simulink model "TST_Rail_MonMeUn"  (R2016b)
settings: Solver=FixedStepDiscrete  StartTime=0.0  StopTime=simTime  FixedStep=sampleTime  RelTol=1e-3
values from neighbouring files (symbols this model uses):
  testCase = 1    [initTST_Rail_MonMeUn_001.m]    (also in initTST_Rail_MonMeUn_002.m = 2; initTST_Rail_MonMeUn_003.m = 3; initTST_Rail_MonMeUn_004.m = 4; initTST_Rail_MonMeUn_005.m = 5)
libraries: simulink x91, UnitTest_Lib x81
(part 4 of 5)

== system TST_Rail_MonMeUn/simulationInput/testSignals_R005 ==
  BC : BusCreator  Inputs=40
  spec_APP_r : FromWorkspace  VariableName=testSig_APP_r  Interpolate=off  OutputAfterFinalValue=Holding final value
  spec_DFC_RailMeUn0_DSM : FromWorkspace  VariableName=testSig_DFC_RailMeUn0_DSM  Interpolate=off  OutputAfterFinalValue=Holding final value
  spec_DFC_RailMeUn10_DSM : FromWorkspace  VariableName=testSig_DFC_RailMeUn10_DSM  Interpolate=off  OutputAfterFinalValue=Holding final value
  spec_DFC_RailMeUn22_DSM : FromWorkspace  VariableName=testSig_DFC_RailMeUn22_DSM  Interpolate=off  OutputAfterFinalValue=Holding final value
  spec_DFC_RailMeUn2_DSM : FromWorkspace  VariableName=testSig_DFC_RailMeUn2_DSM  Interpolate=off  OutputAfterFinalValue=Holding final value
  spec_DFC_RailMeUn3_DSM : FromWorkspace  VariableName=testSig_DFC_RailMeUn3_DSM  Interpolate=off  OutputAfterFinalValue=Holding final value
  spec_DFC_RailMeUn42_DSM : FromWorkspace  VariableName=testSig_DFC_RailMeUn42_DSM  Interpolate=off  OutputAfterFinalValue=Holding final value
  spec_DFC_RailMeUn4_DSM : FromWorkspace  VariableName=testSig_DFC_RailMeUn4_DSM  Interpolate=off  OutputAfterFinalValue=Holding final value
  spec_DFC_RailMeUn7_DSM : FromWorkspace  VariableName=testSig_DFC_RailMeUn7_DSM  Interpolate=off  OutputAfterFinalValue=Holding final value
  spec_DFC_RailMeUn8_DSM : FromWorkspace  VariableName=testSig_DFC_RailMeUn8_DSM  Interpolate=off  OutputAfterFinalValue=Holding final value
  spec_DSM_bRailMeUn0Blk : FromWorkspace  VariableName=testSig_DSM_bRailMeUn0Blk  Interpolate=off  OutputAfterFinalValue=Holding final value
  spec_DSM_bRailMeUn0Rls : FromWorkspace  VariableName=testSig_DSM_bRailMeUn0Rls  Interpolate=off  OutputAfterFinalValue=Holding final value
  spec_DSM_bRailMeUn10Blk : FromWorkspace  VariableName=testSig_DSM_bRailMeUn10Blk  Interpolate=off  OutputAfterFinalValue=Holding final value
  spec_DSM_bRailMeUn10Rls : FromWorkspace  VariableName=testSig_DSM_bRailMeUn10Rls  Interpolate=off  OutputAfterFinalValue=Holding final value
  spec_DSM_bRailMeUn22Blk : FromWorkspace  VariableName=testSig_DSM_bRailMeUn22Blk  Interpolate=off  OutputAfterFinalValue=Holding final value
  spec_DSM_bRailMeUn22Rls : FromWorkspace  VariableName=testSig_DSM_bRailMeUn22Rls  Interpolate=off  OutputAfterFinalValue=Holding final value
  spec_DSM_bRailMeUn2Blk : FromWorkspace  VariableName=testSig_DSM_bRailMeUn2Blk  Interpolate=off  OutputAfterFinalValue=Holding final value
  spec_DSM_bRailMeUn2Rls : FromWorkspace  VariableName=testSig_DSM_bRailMeUn2Rls  Interpolate=off  OutputAfterFinalValue=Holding final value
  spec_DSM_bRailMeUn3Blk : FromWorkspace  VariableName=testSig_DSM_bRailMeUn3Blk  Interpolate=off  OutputAfterFinalValue=Holding final value
  spec_DSM_bRailMeUn3Rls : FromWorkspace  VariableName=testSig_DSM_bRailMeUn3Rls  Interpolate=off  OutputAfterFinalValue=Holding final value
  spec_DSM_bRailMeUn42Blk : FromWorkspace  VariableName=testSig_DSM_bRailMeUn42Blk  Interpolate=off  OutputAfterFinalValue=Holding final value
  spec_DSM_bRailMeUn42Rls : FromWorkspace  VariableName=testSig_DSM_bRailMeUn42Rls  Interpolate=off  OutputAfterFinalValue=Holding final value
  spec_DSM_bRailMeUn4Blk : FromWorkspace  VariableName=testSig_DSM_bRailMeUn4Blk  Interpolate=off  OutputAfterFinalValue=Holding final value
  spec_DSM_bRailMeUn4Rls : FromWorkspace  VariableName=testSig_DSM_bRailMeUn4Rls  Interpolate=off  OutputAfterFinalValue=Holding final value
  spec_DSM_bRailMeUn7Blk : FromWorkspace  VariableName=testSig_DSM_bRailMeUn7Blk  Interpolate=off  OutputAfterFinalValue=Holding final value
  spec_DSM_bRailMeUn7Rls : FromWorkspace  VariableName=testSig_DSM_bRailMeUn7Rls  Interpolate=off  OutputAfterFinalValue=Holding final value
  spec_DSM_bRailMeUn8Blk : FromWorkspace  VariableName=testSig_DSM_bRailMeUn8Blk  Interpolate=off  OutputAfterFinalValue=Holding final value
  spec_DSM_bRailMeUn8Rls : FromWorkspace  VariableName=testSig_DSM_bRailMeUn8Rls  Interpolate=off  OutputAfterFinalValue=Holding final value
  spec_Epm_nEng : FromWorkspace  VariableName=testSig_Epm_nEng  Interpolate=off  OutputAfterFinalValue=Holding final value
  spec_FuelT_tFlSys : FromWorkspace  VariableName=testSig_FuelT_tFlSys  Interpolate=off  OutputAfterFinalValue=Holding final value
  spec_InjCtl_qSetUnBal : FromWorkspace  VariableName=testSig_InjCtl_qSetUnBal  Interpolate=off  OutputAfterFinalValue=Holding final value
  spec_MeUn_dvolSet : FromWorkspace  VariableName=testSig_MeUn_dvolSet  Interpolate=off  OutputAfterFinalValue=Holding final value
  spec_MeUn_dvolSetAdapt : FromWorkspace  VariableName=testSig_MeUn_dvolSetAdapt  Interpolate=off  OutputAfterFinalValue=Holding final value
  spec_PthSet_stOvrRun : FromWorkspace  VariableName=testSig_PthSet_stOvrRun  Interpolate=off  OutputAfterFinalValue=Holding final value
  spec_RailP_pFlt : FromWorkspace  VariableName=testSig_RailP_pFlt  Interpolate=off  OutputAfterFinalValue=Holding final value
  spec_Rail_dvolDemSysMax : FromWorkspace  VariableName=testSig_Rail_dvolDemSysMax  Interpolate=off  OutputAfterFinalValue=Holding final value
  spec_Rail_dvolMeUnCtlUpLim : FromWorkspace  VariableName=testSig_Rail_dvolMeUnCtlUpLim  Interpolate=off  OutputAfterFinalValue=Holding final value
  spec_Rail_pDvt : FromWorkspace  VariableName=testSig_Rail_pDvt  Interpolate=off  OutputAfterFinalValue=Holding final value
  spec_Rail_pSetPoint : FromWorkspace  VariableName=testSig_Rail_pSetPoint  Interpolate=off  OutputAfterFinalValue=Holding final value
  spec_Rail_stCtlLoop : FromWorkspace  VariableName=testSig_Rail_stCtlLoop  Interpolate=off  OutputAfterFinalValue=Holding final value
  testSignals : Outport
  wires:
  BC/1 -> testSignals/1
  spec_Rail_pDvt/1 -> BC/1  "testSig_Rail_pDvt"
  spec_Epm_nEng/1 -> BC/2  "testSig_Epm_nEng"
  spec_MeUn_dvolSet/1 -> BC/3  "testSig_MeUn_dvolSet"
  spec_Rail_dvolMeUnCtlUpLim/1 -> BC/4  "testSig_Rail_dvolMeUnCtlUpLim"
  spec_Rail_stCtlLoop/1 -> BC/5  "testSig_Rail_stCtlLoop"
  spec_InjCtl_qSetUnBal/1 -> BC/6  "testSig_InjCtl_qSetUnBal"
  spec_FuelT_tFlSys/1 -> BC/7  "testSig_FuelT_tFlSys"
  spec_Rail_pSetPoint/1 -> BC/8  "testSig_Rail_pSetPoint"
  spec_Rail_dvolDemSysMax/1 -> BC/9  "testSig_Rail_dvolDemSysMax"
  spec_RailP_pFlt/1 -> BC/10  "testSig_RailP_pFlt"
  spec_MeUn_dvolSetAdapt/1 -> BC/11  "testSig_MeUn_dvolSetAdapt"
  spec_PthSet_stOvrRun/1 -> BC/12  "testSig_PthSet_stOvrRun"
  spec_APP_r/1 -> BC/13  "testSig_APP_r"
  spec_DSM_bRailMeUn0Rls/1 -> BC/14  "testSig_DSM_bRailMeUn0Rls"
  spec_DSM_bRailMeUn0Blk/1 -> BC/15  "testSig_DSM_bRailMeUn0Blk"
  spec_DSM_bRailMeUn2Rls/1 -> BC/16  "testSig_DSM_bRailMeUn2Rls"
  spec_DSM_bRailMeUn2Blk/1 -> BC/17  "testSig_DSM_bRailMeUn2Blk"
  spec_DSM_bRailMeUn22Rls/1 -> BC/18  "testSig_DSM_bRailMeUn22Rls"
  spec_DSM_bRailMeUn22Blk/1 -> BC/19  "testSig_DSM_bRailMeUn22Blk"
  spec_DSM_bRailMeUn3Rls/1 -> BC/20  "testSig_DSM_bRailMeUn3Rls"
  spec_DSM_bRailMeUn3Blk/1 -> BC/21  "testSig_DSM_bRailMeUn3Blk"
  spec_DSM_bRailMeUn4Rls/1 -> BC/22  "testSig_DSM_bRailMeUn4Rls"
  spec_DSM_bRailMeUn4Blk/1 -> BC/23  "testSig_DSM_bRailMeUn4Blk"
  spec_DSM_bRailMeUn42Rls/1 -> BC/24  "testSig_DSM_bRailMeUn42Rls"
  spec_DSM_bRailMeUn42Blk/1 -> BC/25  "testSig_DSM_bRailMeUn42Blk"
  spec_DSM_bRailMeUn7Rls/1 -> BC/26  "testSig_DSM_bRailMeUn7Rls"
  spec_DSM_bRailMeUn7Blk/1 -> BC/27  "testSig_DSM_bRailMeUn7Blk"
  spec_DSM_bRailMeUn8Rls/1 -> BC/28  "testSig_DSM_bRailMeUn8Rls"
  spec_DSM_bRailMeUn8Blk/1 -> BC/29  "testSig_DSM_bRailMeUn8Blk"
  spec_DSM_bRailMeUn10Rls/1 -> BC/30  "testSig_DSM_bRailMeUn10Rls"
  spec_DSM_bRailMeUn10Blk/1 -> BC/31  "testSig_DSM_bRailMeUn10Blk"
  spec_DFC_RailMeUn0_DSM/1 -> BC/32  "testSig_DFC_RailMeUn0_DSM"
  spec_DFC_RailMeUn2_DSM/1 -> BC/33  "testSig_DFC_RailMeUn2_DSM"
  spec_DFC_RailMeUn22_DSM/1 -> BC/34  "testSig_DFC_RailMeUn22_DSM"
  spec_DFC_RailMeUn3_DSM/1 -> BC/35  "testSig_DFC_RailMeUn3_DSM"
  spec_DFC_RailMeUn4_DSM/1 -> BC/36  "testSig_DFC_RailMeUn4_DSM"
  spec_DFC_RailMeUn42_DSM/1 -> BC/37  "testSig_DFC_RailMeUn42_DSM"
  spec_DFC_RailMeUn7_DSM/1 -> BC/38  "testSig_DFC_RailMeUn7_DSM"
  spec_DFC_RailMeUn8_DSM/1 -> BC/39  "testSig_DFC_RailMeUn8_DSM"
  spec_DFC_RailMeUn10_DSM/1 -> BC/40  "testSig_DFC_RailMeUn10_DSM"

== system TST_Rail_MonMeUn/simulationInput/testSignals_R006 ==
  BC : BusCreator  Inputs=40
  spec_APP_r : FromWorkspace  VariableName=testSig_APP_r  Interpolate=off  OutputAfterFinalValue=Holding final value
  spec_DFC_RailMeUn0_DSM : FromWorkspace  VariableName=testSig_DFC_RailMeUn0_DSM  Interpolate=off  OutputAfterFinalValue=Holding final value
  spec_DFC_RailMeUn10_DSM : FromWorkspace  VariableName=testSig_DFC_RailMeUn10_DSM  Interpolate=off  OutputAfterFinalValue=Holding final value
  spec_DFC_RailMeUn22_DSM : FromWorkspace  VariableName=testSig_DFC_RailMeUn22_DSM  Interpolate=off  OutputAfterFinalValue=Holding final value
  spec_DFC_RailMeUn2_DSM : FromWorkspace  VariableName=testSig_DFC_RailMeUn2_DSM  Interpolate=off  OutputAfterFinalValue=Holding final value
  spec_DFC_RailMeUn3_DSM : FromWorkspace  VariableName=testSig_DFC_RailMeUn3_DSM  Interpolate=off  OutputAfterFinalValue=Holding final value
  spec_DFC_RailMeUn42_DSM : FromWorkspace  VariableName=testSig_DFC_RailMeUn42_DSM  Interpolate=off  OutputAfterFinalValue=Holding final value
  spec_DFC_RailMeUn4_DSM : FromWorkspace  VariableName=testSig_DFC_RailMeUn4_DSM  Interpolate=off  OutputAfterFinalValue=Holding final value
  spec_DFC_RailMeUn7_DSM : FromWorkspace  VariableName=testSig_DFC_RailMeUn7_DSM  Interpolate=off  OutputAfterFinalValue=Holding final value
  spec_DFC_RailMeUn8_DSM : FromWorkspace  VariableName=testSig_DFC_RailMeUn8_DSM  Interpolate=off  OutputAfterFinalValue=Holding final value
  spec_DSM_bRailMeUn0Blk : FromWorkspace  VariableName=testSig_DSM_bRailMeUn0Blk  Interpolate=off  OutputAfterFinalValue=Holding final value
  spec_DSM_bRailMeUn0Rls : FromWorkspace  VariableName=testSig_DSM_bRailMeUn0Rls  Interpolate=off  OutputAfterFinalValue=Holding final value
  spec_DSM_bRailMeUn10Blk : FromWorkspace  VariableName=testSig_DSM_bRailMeUn10Blk  Interpolate=off  OutputAfterFinalValue=Holding final value
  spec_DSM_bRailMeUn10Rls : FromWorkspace  VariableName=testSig_DSM_bRailMeUn10Rls  Interpolate=off  OutputAfterFinalValue=Holding final value
  spec_DSM_bRailMeUn22Blk : FromWorkspace  VariableName=testSig_DSM_bRailMeUn22Blk  Interpolate=off  OutputAfterFinalValue=Holding final value
  spec_DSM_bRailMeUn22Rls : FromWorkspace  VariableName=testSig_DSM_bRailMeUn22Rls  Interpolate=off  OutputAfterFinalValue=Holding final value
  spec_DSM_bRailMeUn2Blk : FromWorkspace  VariableName=testSig_DSM_bRailMeUn2Blk  Interpolate=off  OutputAfterFinalValue=Holding final value
  spec_DSM_bRailMeUn2Rls : FromWorkspace  VariableName=testSig_DSM_bRailMeUn2Rls  Interpolate=off  OutputAfterFinalValue=Holding final value
  spec_DSM_bRailMeUn3Blk : FromWorkspace  VariableName=testSig_DSM_bRailMeUn3Blk  Interpolate=off  OutputAfterFinalValue=Holding final value
  spec_DSM_bRailMeUn3Rls : FromWorkspace  VariableName=testSig_DSM_bRailMeUn3Rls  Interpolate=off  OutputAfterFinalValue=Holding final value
  spec_DSM_bRailMeUn42Blk : FromWorkspace  VariableName=testSig_DSM_bRailMeUn42Blk  Interpolate=off  OutputAfterFinalValue=Holding final value
  spec_DSM_bRailMeUn42Rls : FromWorkspace  VariableName=testSig_DSM_bRailMeUn42Rls  Interpolate=off  OutputAfterFinalValue=Holding final value
  spec_DSM_bRailMeUn4Blk : FromWorkspace  VariableName=testSig_DSM_bRailMeUn4Blk  Interpolate=off  OutputAfterFinalValue=Holding final value
  spec_DSM_bRailMeUn4Rls : FromWorkspace  VariableName=testSig_DSM_bRailMeUn4Rls  Interpolate=off  OutputAfterFinalValue=Holding final value
  spec_DSM_bRailMeUn7Blk : FromWorkspace  VariableName=testSig_DSM_bRailMeUn7Blk  Interpolate=off  OutputAfterFinalValue=Holding final value
  spec_DSM_bRailMeUn7Rls : FromWorkspace  VariableName=testSig_DSM_bRailMeUn7Rls  Interpolate=off  OutputAfterFinalValue=Holding final value
  spec_DSM_bRailMeUn8Blk : FromWorkspace  VariableName=testSig_DSM_bRailMeUn8Blk  Interpolate=off  OutputAfterFinalValue=Holding final value
  spec_DSM_bRailMeUn8Rls : FromWorkspace  VariableName=testSig_DSM_bRailMeUn8Rls  Interpolate=off  OutputAfterFinalValue=Holding final value
  spec_Epm_nEng : FromWorkspace  VariableName=testSig_Epm_nEng  Interpolate=off  OutputAfterFinalValue=Holding final value
  spec_FuelT_tFlSys : FromWorkspace  VariableName=testSig_FuelT_tFlSys  Interpolate=off  OutputAfterFinalValue=Holding final value
  spec_InjCtl_qSetUnBal : FromWorkspace  VariableName=testSig_InjCtl_qSetUnBal  Interpolate=off  OutputAfterFinalValue=Holding final value
  spec_MeUn_dvolSet : FromWorkspace  VariableName=testSig_MeUn_dvolSet  Interpolate=off  OutputAfterFinalValue=Holding final value
  spec_MeUn_dvolSetAdapt : FromWorkspace  VariableName=testSig_MeUn_dvolSetAdapt  Interpolate=off  OutputAfterFinalValue=Holding final value
  spec_PthSet_stOvrRun : FromWorkspace  VariableName=testSig_PthSet_stOvrRun  Interpolate=off  OutputAfterFinalValue=Holding final value
  spec_RailP_pFlt : FromWorkspace  VariableName=testSig_RailP_pFlt  Interpolate=off  OutputAfterFinalValue=Holding final value
  spec_Rail_dvolDemSysMax : FromWorkspace  VariableName=testSig_Rail_dvolDemSysMax  Interpolate=off  OutputAfterFinalValue=Holding final value
  spec_Rail_dvolMeUnCtlUpLim : FromWorkspace  VariableName=testSig_Rail_dvolMeUnCtlUpLim  Interpolate=off  OutputAfterFinalValue=Holding final value
  spec_Rail_pDvt : FromWorkspace  VariableName=testSig_Rail_pDvt  Interpolate=off  OutputAfterFinalValue=Holding final value
  spec_Rail_pSetPoint : FromWorkspace  VariableName=testSig_Rail_pSetPoint  Interpolate=off  OutputAfterFinalValue=Holding final value
  spec_Rail_stCtlLoop : FromWorkspace  VariableName=testSig_Rail_stCtlLoop  Interpolate=off  OutputAfterFinalValue=Holding final value
  testSignals : Outport
  wires:
  BC/1 -> testSignals/1
  spec_Rail_pDvt/1 -> BC/1  "testSig_Rail_pDvt"
  spec_Epm_nEng/1 -> BC/2  "testSig_Epm_nEng"
  spec_MeUn_dvolSet/1 -> BC/3  "testSig_MeUn_dvolSet"
  spec_Rail_dvolMeUnCtlUpLim/1 -> BC/4  "testSig_Rail_dvolMeUnCtlUpLim"
  spec_Rail_stCtlLoop/1 -> BC/5  "testSig_Rail_stCtlLoop"
  spec_InjCtl_qSetUnBal/1 -> BC/6  "testSig_InjCtl_qSetUnBal"
  spec_FuelT_tFlSys/1 -> BC/7  "testSig_FuelT_tFlSys"
  spec_Rail_pSetPoint/1 -> BC/8  "testSig_Rail_pSetPoint"
  spec_Rail_dvolDemSysMax/1 -> BC/9  "testSig_Rail_dvolDemSysMax"
  spec_RailP_pFlt/1 -> BC/10  "testSig_RailP_pFlt"
  spec_MeUn_dvolSetAdapt/1 -> BC/11  "testSig_MeUn_dvolSetAdapt"
  spec_PthSet_stOvrRun/1 -> BC/12  "testSig_PthSet_stOvrRun"
  spec_APP_r/1 -> BC/13  "testSig_APP_r"
  spec_DSM_bRailMeUn0Rls/1 -> BC/14  "testSig_DSM_bRailMeUn0Rls"
  spec_DSM_bRailMeUn0Blk/1 -> BC/15  "testSig_DSM_bRailMeUn0Blk"
  spec_DSM_bRailMeUn2Rls/1 -> BC/16  "testSig_DSM_bRailMeUn2Rls"
  spec_DSM_bRailMeUn2Blk/1 -> BC/17  "testSig_DSM_bRailMeUn2Blk"
  spec_DSM_bRailMeUn22Rls/1 -> BC/18  "testSig_DSM_bRailMeUn22Rls"
  spec_DSM_bRailMeUn22Blk/1 -> BC/19  "testSig_DSM_bRailMeUn22Blk"
  spec_DSM_bRailMeUn3Rls/1 -> BC/20  "testSig_DSM_bRailMeUn3Rls"
  spec_DSM_bRailMeUn3Blk/1 -> BC/21  "testSig_DSM_bRailMeUn3Blk"
  spec_DSM_bRailMeUn4Rls/1 -> BC/22  "testSig_DSM_bRailMeUn4Rls"
  spec_DSM_bRailMeUn4Blk/1 -> BC/23  "testSig_DSM_bRailMeUn4Blk"
  spec_DSM_bRailMeUn42Rls/1 -> BC/24  "testSig_DSM_bRailMeUn42Rls"
  spec_DSM_bRailMeUn42Blk/1 -> BC/25  "testSig_DSM_bRailMeUn42Blk"
  spec_DSM_bRailMeUn7Rls/1 -> BC/26  "testSig_DSM_bRailMeUn7Rls"
  spec_DSM_bRailMeUn7Blk/1 -> BC/27  "testSig_DSM_bRailMeUn7Blk"
  spec_DSM_bRailMeUn8Rls/1 -> BC/28  "testSig_DSM_bRailMeUn8Rls"
  spec_DSM_bRailMeUn8Blk/1 -> BC/29  "testSig_DSM_bRailMeUn8Blk"
  spec_DSM_bRailMeUn10Rls/1 -> BC/30  "testSig_DSM_bRailMeUn10Rls"
  spec_DSM_bRailMeUn10Blk/1 -> BC/31  "testSig_DSM_bRailMeUn10Blk"
  spec_DFC_RailMeUn0_DSM/1 -> BC/32  "testSig_DFC_RailMeUn0_DSM"
  spec_DFC_RailMeUn2_DSM/1 -> BC/33  "testSig_DFC_RailMeUn2_DSM"
  spec_DFC_RailMeUn22_DSM/1 -> BC/34  "testSig_DFC_RailMeUn22_DSM"
  spec_DFC_RailMeUn3_DSM/1 -> BC/35  "testSig_DFC_RailMeUn3_DSM"
  spec_DFC_RailMeUn4_DSM/1 -> BC/36  "testSig_DFC_RailMeUn4_DSM"
  spec_DFC_RailMeUn42_DSM/1 -> BC/37  "testSig_DFC_RailMeUn42_DSM"
  spec_DFC_RailMeUn7_DSM/1 -> BC/38  "testSig_DFC_RailMeUn7_DSM"
  spec_DFC_RailMeUn8_DSM/1 -> BC/39  "testSig_DFC_RailMeUn8_DSM"
  spec_DFC_RailMeUn10_DSM/1 -> BC/40  "testSig_DFC_RailMeUn10_DSM"

== system TST_Rail_MonMeUn/simulationInput/testSignals_R007 ==
  BC : BusCreator  Inputs=40
  spec_APP_r : FromWorkspace  VariableName=testSig_APP_r  Interpolate=off  OutputAfterFinalValue=Holding final value
  spec_DFC_RailMeUn0_DSM : FromWorkspace  VariableName=testSig_DFC_RailMeUn0_DSM  Interpolate=off  OutputAfterFinalValue=Holding final value
  spec_DFC_RailMeUn10_DSM : FromWorkspace  VariableName=testSig_DFC_RailMeUn10_DSM  Interpolate=off  OutputAfterFinalValue=Holding final value
  spec_DFC_RailMeUn22_DSM : FromWorkspace  VariableName=testSig_DFC_RailMeUn22_DSM  Interpolate=off  OutputAfterFinalValue=Holding final value
  spec_DFC_RailMeUn2_DSM : FromWorkspace  VariableName=testSig_DFC_RailMeUn2_DSM  Interpolate=off  OutputAfterFinalValue=Holding final value
  spec_DFC_RailMeUn3_DSM : FromWorkspace  VariableName=testSig_DFC_RailMeUn3_DSM  Interpolate=off  OutputAfterFinalValue=Holding final value
  spec_DFC_RailMeUn42_DSM : FromWorkspace  VariableName=testSig_DFC_RailMeUn42_DSM  Interpolate=off  OutputAfterFinalValue=Holding final value
  spec_DFC_RailMeUn4_DSM : FromWorkspace  VariableName=testSig_DFC_RailMeUn4_DSM  Interpolate=off  OutputAfterFinalValue=Holding final value
  spec_DFC_RailMeUn7_DSM : FromWorkspace  VariableName=testSig_DFC_RailMeUn7_DSM  Interpolate=off  OutputAfterFinalValue=Holding final value
  spec_DFC_RailMeUn8_DSM : FromWorkspace  VariableName=testSig_DFC_RailMeUn8_DSM  Interpolate=off  OutputAfterFinalValue=Holding final value
  spec_DSM_bRailMeUn0Blk : FromWorkspace  VariableName=testSig_DSM_bRailMeUn0Blk  Interpolate=off  OutputAfterFinalValue=Holding final value
  spec_DSM_bRailMeUn0Rls : FromWorkspace  VariableName=testSig_DSM_bRailMeUn0Rls  Interpolate=off  OutputAfterFinalValue=Holding final value
  spec_DSM_bRailMeUn10Blk : FromWorkspace  VariableName=testSig_DSM_bRailMeUn10Blk  Interpolate=off  OutputAfterFinalValue=Holding final value
  spec_DSM_bRailMeUn10Rls : FromWorkspace  VariableName=testSig_DSM_bRailMeUn10Rls  Interpolate=off  OutputAfterFinalValue=Holding final value
  spec_DSM_bRailMeUn22Blk : FromWorkspace  VariableName=testSig_DSM_bRailMeUn22Blk  Interpolate=off  OutputAfterFinalValue=Holding final value
  spec_DSM_bRailMeUn22Rls : FromWorkspace  VariableName=testSig_DSM_bRailMeUn22Rls  Interpolate=off  OutputAfterFinalValue=Holding final value
  spec_DSM_bRailMeUn2Blk : FromWorkspace  VariableName=testSig_DSM_bRailMeUn2Blk  Interpolate=off  OutputAfterFinalValue=Holding final value
  spec_DSM_bRailMeUn2Rls : FromWorkspace  VariableName=testSig_DSM_bRailMeUn2Rls  Interpolate=off  OutputAfterFinalValue=Holding final value
  spec_DSM_bRailMeUn3Blk : FromWorkspace  VariableName=testSig_DSM_bRailMeUn3Blk  Interpolate=off  OutputAfterFinalValue=Holding final value
  spec_DSM_bRailMeUn3Rls : FromWorkspace  VariableName=testSig_DSM_bRailMeUn3Rls  Interpolate=off  OutputAfterFinalValue=Holding final value
  spec_DSM_bRailMeUn42Blk : FromWorkspace  VariableName=testSig_DSM_bRailMeUn42Blk  Interpolate=off  OutputAfterFinalValue=Holding final value
  spec_DSM_bRailMeUn42Rls : FromWorkspace  VariableName=testSig_DSM_bRailMeUn42Rls  Interpolate=off  OutputAfterFinalValue=Holding final value
  spec_DSM_bRailMeUn4Blk : FromWorkspace  VariableName=testSig_DSM_bRailMeUn4Blk  Interpolate=off  OutputAfterFinalValue=Holding final value
  spec_DSM_bRailMeUn4Rls : FromWorkspace  VariableName=testSig_DSM_bRailMeUn4Rls  Interpolate=off  OutputAfterFinalValue=Holding final value
  spec_DSM_bRailMeUn7Blk : FromWorkspace  VariableName=testSig_DSM_bRailMeUn7Blk  Interpolate=off  OutputAfterFinalValue=Holding final value
  spec_DSM_bRailMeUn7Rls : FromWorkspace  VariableName=testSig_DSM_bRailMeUn7Rls  Interpolate=off  OutputAfterFinalValue=Holding final value
  spec_DSM_bRailMeUn8Blk : FromWorkspace  VariableName=testSig_DSM_bRailMeUn8Blk  Interpolate=off  OutputAfterFinalValue=Holding final value
  spec_DSM_bRailMeUn8Rls : FromWorkspace  VariableName=testSig_DSM_bRailMeUn8Rls  Interpolate=off  OutputAfterFinalValue=Holding final value
  spec_Epm_nEng : FromWorkspace  VariableName=testSig_Epm_nEng  Interpolate=off  OutputAfterFinalValue=Holding final value
  spec_FuelT_tFlSys : FromWorkspace  VariableName=testSig_FuelT_tFlSys  Interpolate=off  OutputAfterFinalValue=Holding final value
  spec_InjCtl_qSetUnBal : FromWorkspace  VariableName=testSig_InjCtl_qSetUnBal  Interpolate=off  OutputAfterFinalValue=Holding final value
  spec_MeUn_dvolSet : FromWorkspace  VariableName=testSig_MeUn_dvolSet  Interpolate=off  OutputAfterFinalValue=Holding final value
  spec_MeUn_dvolSetAdapt : FromWorkspace  VariableName=testSig_MeUn_dvolSetAdapt  Interpolate=off  OutputAfterFinalValue=Holding final value
  spec_PthSet_stOvrRun : FromWorkspace  VariableName=testSig_PthSet_stOvrRun  Interpolate=off  OutputAfterFinalValue=Holding final value
  spec_RailP_pFlt : FromWorkspace  VariableName=testSig_RailP_pFlt  Interpolate=off  OutputAfterFinalValue=Holding final value
  spec_Rail_dvolDemSysMax : FromWorkspace  VariableName=testSig_Rail_dvolDemSysMax  Interpolate=off  OutputAfterFinalValue=Holding final value
  spec_Rail_dvolMeUnCtlUpLim : FromWorkspace  VariableName=testSig_Rail_dvolMeUnCtlUpLim  Interpolate=off  OutputAfterFinalValue=Holding final value
  spec_Rail_pDvt : FromWorkspace  VariableName=testSig_Rail_pDvt  Interpolate=off  OutputAfterFinalValue=Holding final value
  spec_Rail_pSetPoint : FromWorkspace  VariableName=testSig_Rail_pSetPoint  Interpolate=off  OutputAfterFinalValue=Holding final value
  spec_Rail_stCtlLoop : FromWorkspace  VariableName=testSig_Rail_stCtlLoop  Interpolate=off  OutputAfterFinalValue=Holding final value
  testSignals : Outport
  wires:
  BC/1 -> testSignals/1
  spec_Rail_pDvt/1 -> BC/1  "testSig_Rail_pDvt"
  spec_Epm_nEng/1 -> BC/2  "testSig_Epm_nEng"
  spec_MeUn_dvolSet/1 -> BC/3  "testSig_MeUn_dvolSet"
  spec_Rail_dvolMeUnCtlUpLim/1 -> BC/4  "testSig_Rail_dvolMeUnCtlUpLim"
  spec_Rail_stCtlLoop/1 -> BC/5  "testSig_Rail_stCtlLoop"
  spec_InjCtl_qSetUnBal/1 -> BC/6  "testSig_InjCtl_qSetUnBal"
  spec_FuelT_tFlSys/1 -> BC/7  "testSig_FuelT_tFlSys"
  spec_Rail_pSetPoint/1 -> BC/8  "testSig_Rail_pSetPoint"
  spec_Rail_dvolDemSysMax/1 -> BC/9  "testSig_Rail_dvolDemSysMax"
  spec_RailP_pFlt/1 -> BC/10  "testSig_RailP_pFlt"
  spec_MeUn_dvolSetAdapt/1 -> BC/11  "testSig_MeUn_dvolSetAdapt"
  spec_PthSet_stOvrRun/1 -> BC/12  "testSig_PthSet_stOvrRun"
  spec_APP_r/1 -> BC/13  "testSig_APP_r"
  spec_DSM_bRailMeUn0Rls/1 -> BC/14  "testSig_DSM_bRailMeUn0Rls"
  spec_DSM_bRailMeUn0Blk/1 -> BC/15  "testSig_DSM_bRailMeUn0Blk"
  spec_DSM_bRailMeUn2Rls/1 -> BC/16  "testSig_DSM_bRailMeUn2Rls"
  spec_DSM_bRailMeUn2Blk/1 -> BC/17  "testSig_DSM_bRailMeUn2Blk"
  spec_DSM_bRailMeUn22Rls/1 -> BC/18  "testSig_DSM_bRailMeUn22Rls"
  spec_DSM_bRailMeUn22Blk/1 -> BC/19  "testSig_DSM_bRailMeUn22Blk"
  spec_DSM_bRailMeUn3Rls/1 -> BC/20  "testSig_DSM_bRailMeUn3Rls"
  spec_DSM_bRailMeUn3Blk/1 -> BC/21  "testSig_DSM_bRailMeUn3Blk"
  spec_DSM_bRailMeUn4Rls/1 -> BC/22  "testSig_DSM_bRailMeUn4Rls"
  spec_DSM_bRailMeUn4Blk/1 -> BC/23  "testSig_DSM_bRailMeUn4Blk"
  spec_DSM_bRailMeUn42Rls/1 -> BC/24  "testSig_DSM_bRailMeUn42Rls"
  spec_DSM_bRailMeUn42Blk/1 -> BC/25  "testSig_DSM_bRailMeUn42Blk"
  spec_DSM_bRailMeUn7Rls/1 -> BC/26  "testSig_DSM_bRailMeUn7Rls"
  spec_DSM_bRailMeUn7Blk/1 -> BC/27  "testSig_DSM_bRailMeUn7Blk"
  spec_DSM_bRailMeUn8Rls/1 -> BC/28  "testSig_DSM_bRailMeUn8Rls"
  spec_DSM_bRailMeUn8Blk/1 -> BC/29  "testSig_DSM_bRailMeUn8Blk"
  spec_DSM_bRailMeUn10Rls/1 -> BC/30  "testSig_DSM_bRailMeUn10Rls"
  spec_DSM_bRailMeUn10Blk/1 -> BC/31  "testSig_DSM_bRailMeUn10Blk"
  spec_DFC_RailMeUn0_DSM/1 -> BC/32  "testSig_DFC_RailMeUn0_DSM"
  spec_DFC_RailMeUn2_DSM/1 -> BC/33  "testSig_DFC_RailMeUn2_DSM"
  spec_DFC_RailMeUn22_DSM/1 -> BC/34  "testSig_DFC_RailMeUn22_DSM"
  spec_DFC_RailMeUn3_DSM/1 -> BC/35  "testSig_DFC_RailMeUn3_DSM"
  spec_DFC_RailMeUn4_DSM/1 -> BC/36  "testSig_DFC_RailMeUn4_DSM"
  spec_DFC_RailMeUn42_DSM/1 -> BC/37  "testSig_DFC_RailMeUn42_DSM"
  spec_DFC_RailMeUn7_DSM/1 -> BC/38  "testSig_DFC_RailMeUn7_DSM"
  spec_DFC_RailMeUn8_DSM/1 -> BC/39  "testSig_DFC_RailMeUn8_DSM"
  spec_DFC_RailMeUn10_DSM/1 -> BC/40  "testSig_DFC_RailMeUn10_DSM"

== system TST_Rail_MonMeUn/simulationInput/testSignals_R008 ==
  BC : BusCreator  Inputs=40
  spec_APP_r : FromWorkspace  VariableName=testSig_APP_r  Interpolate=off  OutputAfterFinalValue=Holding final value
  spec_DFC_RailMeUn0_DSM : FromWorkspace  VariableName=testSig_DFC_RailMeUn0_DSM  Interpolate=off  OutputAfterFinalValue=Holding final value
  spec_DFC_RailMeUn10_DSM : FromWorkspace  VariableName=testSig_DFC_RailMeUn10_DSM  Interpolate=off  OutputAfterFinalValue=Holding final value
  spec_DFC_RailMeUn22_DSM : FromWorkspace  VariableName=testSig_DFC_RailMeUn22_DSM  Interpolate=off  OutputAfterFinalValue=Holding final value
  spec_DFC_RailMeUn2_DSM : FromWorkspace  VariableName=testSig_DFC_RailMeUn2_DSM  Interpolate=off  OutputAfterFinalValue=Holding final value
  spec_DFC_RailMeUn3_DSM : FromWorkspace  VariableName=testSig_DFC_RailMeUn3_DSM  Interpolate=off  OutputAfterFinalValue=Holding final value
  spec_DFC_RailMeUn42_DSM : FromWorkspace  VariableName=testSig_DFC_RailMeUn42_DSM  Interpolate=off  OutputAfterFinalValue=Holding final value
  spec_DFC_RailMeUn4_DSM : FromWorkspace  VariableName=testSig_DFC_RailMeUn4_DSM  Interpolate=off  OutputAfterFinalValue=Holding final value
  spec_DFC_RailMeUn7_DSM : FromWorkspace  VariableName=testSig_DFC_RailMeUn7_DSM  Interpolate=off  OutputAfterFinalValue=Holding final value
  spec_DFC_RailMeUn8_DSM : FromWorkspace  VariableName=testSig_DFC_RailMeUn8_DSM  Interpolate=off  OutputAfterFinalValue=Holding final value
  spec_DSM_bRailMeUn0Blk : FromWorkspace  VariableName=testSig_DSM_bRailMeUn0Blk  Interpolate=off  OutputAfterFinalValue=Holding final value
  spec_DSM_bRailMeUn0Rls : FromWorkspace  VariableName=testSig_DSM_bRailMeUn0Rls  Interpolate=off  OutputAfterFinalValue=Holding final value
  spec_DSM_bRailMeUn10Blk : FromWorkspace  VariableName=testSig_DSM_bRailMeUn10Blk  Interpolate=off  OutputAfterFinalValue=Holding final value
  spec_DSM_bRailMeUn10Rls : FromWorkspace  VariableName=testSig_DSM_bRailMeUn10Rls  Interpolate=off  OutputAfterFinalValue=Holding final value
  spec_DSM_bRailMeUn22Blk : FromWorkspace  VariableName=testSig_DSM_bRailMeUn22Blk  Interpolate=off  OutputAfterFinalValue=Holding final value
  spec_DSM_bRailMeUn22Rls : FromWorkspace  VariableName=testSig_DSM_bRailMeUn22Rls  Interpolate=off  OutputAfterFinalValue=Holding final value
  spec_DSM_bRailMeUn2Blk : FromWorkspace  VariableName=testSig_DSM_bRailMeUn2Blk  Interpolate=off  OutputAfterFinalValue=Holding final value
  spec_DSM_bRailMeUn2Rls : FromWorkspace  VariableName=testSig_DSM_bRailMeUn2Rls  Interpolate=off  OutputAfterFinalValue=Holding final value
  spec_DSM_bRailMeUn3Blk : FromWorkspace  VariableName=testSig_DSM_bRailMeUn3Blk  Interpolate=off  OutputAfterFinalValue=Holding final value
  spec_DSM_bRailMeUn3Rls : FromWorkspace  VariableName=testSig_DSM_bRailMeUn3Rls  Interpolate=off  OutputAfterFinalValue=Holding final value
  spec_DSM_bRailMeUn42Blk : FromWorkspace  VariableName=testSig_DSM_bRailMeUn42Blk  Interpolate=off  OutputAfterFinalValue=Holding final value
  spec_DSM_bRailMeUn42Rls : FromWorkspace  VariableName=testSig_DSM_bRailMeUn42Rls  Interpolate=off  OutputAfterFinalValue=Holding final value
  spec_DSM_bRailMeUn4Blk : FromWorkspace  VariableName=testSig_DSM_bRailMeUn4Blk  Interpolate=off  OutputAfterFinalValue=Holding final value
  spec_DSM_bRailMeUn4Rls : FromWorkspace  VariableName=testSig_DSM_bRailMeUn4Rls  Interpolate=off  OutputAfterFinalValue=Holding final value
  spec_DSM_bRailMeUn7Blk : FromWorkspace  VariableName=testSig_DSM_bRailMeUn7Blk  Interpolate=off  OutputAfterFinalValue=Holding final value
  spec_DSM_bRailMeUn7Rls : FromWorkspace  VariableName=testSig_DSM_bRailMeUn7Rls  Interpolate=off  OutputAfterFinalValue=Holding final value
  spec_DSM_bRailMeUn8Blk : FromWorkspace  VariableName=testSig_DSM_bRailMeUn8Blk  Interpolate=off  OutputAfterFinalValue=Holding final value
  spec_DSM_bRailMeUn8Rls : FromWorkspace  VariableName=testSig_DSM_bRailMeUn8Rls  Interpolate=off  OutputAfterFinalValue=Holding final value
  spec_Epm_nEng : FromWorkspace  VariableName=testSig_Epm_nEng  Interpolate=off  OutputAfterFinalValue=Holding final value
  spec_FuelT_tFlSys : FromWorkspace  VariableName=testSig_FuelT_tFlSys  Interpolate=off  OutputAfterFinalValue=Holding final value
  spec_InjCtl_qSetUnBal : FromWorkspace  VariableName=testSig_InjCtl_qSetUnBal  Interpolate=off  OutputAfterFinalValue=Holding final value
  spec_MeUn_dvolSet : FromWorkspace  VariableName=testSig_MeUn_dvolSet  Interpolate=off  OutputAfterFinalValue=Holding final value
  spec_MeUn_dvolSetAdapt : FromWorkspace  VariableName=testSig_MeUn_dvolSetAdapt  Interpolate=off  OutputAfterFinalValue=Holding final value
  spec_PthSet_stOvrRun : FromWorkspace  VariableName=testSig_PthSet_stOvrRun  Interpolate=off  OutputAfterFinalValue=Holding final value
  spec_RailP_pFlt : FromWorkspace  VariableName=testSig_RailP_pFlt  Interpolate=off  OutputAfterFinalValue=Holding final value
  spec_Rail_dvolDemSysMax : FromWorkspace  VariableName=testSig_Rail_dvolDemSysMax  Interpolate=off  OutputAfterFinalValue=Holding final value
  spec_Rail_dvolMeUnCtlUpLim : FromWorkspace  VariableName=testSig_Rail_dvolMeUnCtlUpLim  Interpolate=off  OutputAfterFinalValue=Holding final value
  spec_Rail_pDvt : FromWorkspace  VariableName=testSig_Rail_pDvt  Interpolate=off  OutputAfterFinalValue=Holding final value
  spec_Rail_pSetPoint : FromWorkspace  VariableName=testSig_Rail_pSetPoint  Interpolate=off  OutputAfterFinalValue=Holding final value
  spec_Rail_stCtlLoop : FromWorkspace  VariableName=testSig_Rail_stCtlLoop  Interpolate=off  OutputAfterFinalValue=Holding final value
  testSignals : Outport
  wires:
  BC/1 -> testSignals/1
  spec_Rail_pDvt/1 -> BC/1  "testSig_Rail_pDvt"
  spec_Epm_nEng/1 -> BC/2  "testSig_Epm_nEng"
  spec_MeUn_dvolSet/1 -> BC/3  "testSig_MeUn_dvolSet"
  spec_Rail_dvolMeUnCtlUpLim/1 -> BC/4  "testSig_Rail_dvolMeUnCtlUpLim"
  spec_Rail_stCtlLoop/1 -> BC/5  "testSig_Rail_stCtlLoop"
  spec_InjCtl_qSetUnBal/1 -> BC/6  "testSig_InjCtl_qSetUnBal"
  spec_FuelT_tFlSys/1 -> BC/7  "testSig_FuelT_tFlSys"
  spec_Rail_pSetPoint/1 -> BC/8  "testSig_Rail_pSetPoint"
  spec_Rail_dvolDemSysMax/1 -> BC/9  "testSig_Rail_dvolDemSysMax"
  spec_RailP_pFlt/1 -> BC/10  "testSig_RailP_pFlt"
  spec_MeUn_dvolSetAdapt/1 -> BC/11  "testSig_MeUn_dvolSetAdapt"
  spec_PthSet_stOvrRun/1 -> BC/12  "testSig_PthSet_stOvrRun"
  spec_APP_r/1 -> BC/13  "testSig_APP_r"
  spec_DSM_bRailMeUn0Rls/1 -> BC/14  "testSig_DSM_bRailMeUn0Rls"
  spec_DSM_bRailMeUn0Blk/1 -> BC/15  "testSig_DSM_bRailMeUn0Blk"
  spec_DSM_bRailMeUn2Rls/1 -> BC/16  "testSig_DSM_bRailMeUn2Rls"
  spec_DSM_bRailMeUn2Blk/1 -> BC/17  "testSig_DSM_bRailMeUn2Blk"
  spec_DSM_bRailMeUn22Rls/1 -> BC/18  "testSig_DSM_bRailMeUn22Rls"
  spec_DSM_bRailMeUn22Blk/1 -> BC/19  "testSig_DSM_bRailMeUn22Blk"
  spec_DSM_bRailMeUn3Rls/1 -> BC/20  "testSig_DSM_bRailMeUn3Rls"
  spec_DSM_bRailMeUn3Blk/1 -> BC/21  "testSig_DSM_bRailMeUn3Blk"
  spec_DSM_bRailMeUn4Rls/1 -> BC/22  "testSig_DSM_bRailMeUn4Rls"
  spec_DSM_bRailMeUn4Blk/1 -> BC/23  "testSig_DSM_bRailMeUn4Blk"
  spec_DSM_bRailMeUn42Rls/1 -> BC/24  "testSig_DSM_bRailMeUn42Rls"
  spec_DSM_bRailMeUn42Blk/1 -> BC/25  "testSig_DSM_bRailMeUn42Blk"
  spec_DSM_bRailMeUn7Rls/1 -> BC/26  "testSig_DSM_bRailMeUn7Rls"
  spec_DSM_bRailMeUn7Blk/1 -> BC/27  "testSig_DSM_bRailMeUn7Blk"
  spec_DSM_bRailMeUn8Rls/1 -> BC/28  "testSig_DSM_bRailMeUn8Rls"
  spec_DSM_bRailMeUn8Blk/1 -> BC/29  "testSig_DSM_bRailMeUn8Blk"
  spec_DSM_bRailMeUn10Rls/1 -> BC/30  "testSig_DSM_bRailMeUn10Rls"
  spec_DSM_bRailMeUn10Blk/1 -> BC/31  "testSig_DSM_bRailMeUn10Blk"
  spec_DFC_RailMeUn0_DSM/1 -> BC/32  "testSig_DFC_RailMeUn0_DSM"
  spec_DFC_RailMeUn2_DSM/1 -> BC/33  "testSig_DFC_RailMeUn2_DSM"
  spec_DFC_RailMeUn22_DSM/1 -> BC/34  "testSig_DFC_RailMeUn22_DSM"
  spec_DFC_RailMeUn3_DSM/1 -> BC/35  "testSig_DFC_RailMeUn3_DSM"
  spec_DFC_RailMeUn4_DSM/1 -> BC/36  "testSig_DFC_RailMeUn4_DSM"
  spec_DFC_RailMeUn42_DSM/1 -> BC/37  "testSig_DFC_RailMeUn42_DSM"
  spec_DFC_RailMeUn7_DSM/1 -> BC/38  "testSig_DFC_RailMeUn7_DSM"
  spec_DFC_RailMeUn8_DSM/1 -> BC/39  "testSig_DFC_RailMeUn8_DSM"
  spec_DFC_RailMeUn10_DSM/1 -> BC/40  "testSig_DFC_RailMeUn10_DSM"

== system TST_Rail_MonMeUn/simulationInput/testSignals_R009 ==
  BC : BusCreator  Inputs=40
  spec_APP_r : FromWorkspace  VariableName=testSig_APP_r  Interpolate=off  OutputAfterFinalValue=Holding final value
  spec_DFC_RailMeUn0_DSM : FromWorkspace  VariableName=testSig_DFC_RailMeUn0_DSM  Interpolate=off  OutputAfterFinalValue=Holding final value
  spec_DFC_RailMeUn10_DSM : FromWorkspace  VariableName=testSig_DFC_RailMeUn10_DSM  Interpolate=off  OutputAfterFinalValue=Holding final value
  spec_DFC_RailMeUn22_DSM : FromWorkspace  VariableName=testSig_DFC_RailMeUn22_DSM  Interpolate=off  OutputAfterFinalValue=Holding final value
  spec_DFC_RailMeUn2_DSM : FromWorkspace  VariableName=testSig_DFC_RailMeUn2_DSM  Interpolate=off  OutputAfterFinalValue=Holding final value
  spec_DFC_RailMeUn3_DSM : FromWorkspace  VariableName=testSig_DFC_RailMeUn3_DSM  Interpolate=off  OutputAfterFinalValue=Holding final value
  spec_DFC_RailMeUn42_DSM : FromWorkspace  VariableName=testSig_DFC_RailMeUn42_DSM  Interpolate=off  OutputAfterFinalValue=Holding final value
  spec_DFC_RailMeUn4_DSM : FromWorkspace  VariableName=testSig_DFC_RailMeUn4_DSM  Interpolate=off  OutputAfterFinalValue=Holding final value
  spec_DFC_RailMeUn7_DSM : FromWorkspace  VariableName=testSig_DFC_RailMeUn7_DSM  Interpolate=off  OutputAfterFinalValue=Holding final value
  spec_DFC_RailMeUn8_DSM : FromWorkspace  VariableName=testSig_DFC_RailMeUn8_DSM  Interpolate=off  OutputAfterFinalValue=Holding final value
  spec_DSM_bRailMeUn0Blk : FromWorkspace  VariableName=testSig_DSM_bRailMeUn0Blk  Interpolate=off  OutputAfterFinalValue=Holding final value
  spec_DSM_bRailMeUn0Rls : FromWorkspace  VariableName=testSig_DSM_bRailMeUn0Rls  Interpolate=off  OutputAfterFinalValue=Holding final value
  spec_DSM_bRailMeUn10Blk : FromWorkspace  VariableName=testSig_DSM_bRailMeUn10Blk  Interpolate=off  OutputAfterFinalValue=Holding final value
  spec_DSM_bRailMeUn10Rls : FromWorkspace  VariableName=testSig_DSM_bRailMeUn10Rls  Interpolate=off  OutputAfterFinalValue=Holding final value
  spec_DSM_bRailMeUn22Blk : FromWorkspace  VariableName=testSig_DSM_bRailMeUn22Blk  Interpolate=off  OutputAfterFinalValue=Holding final value
  spec_DSM_bRailMeUn22Rls : FromWorkspace  VariableName=testSig_DSM_bRailMeUn22Rls  Interpolate=off  OutputAfterFinalValue=Holding final value
  spec_DSM_bRailMeUn2Blk : FromWorkspace  VariableName=testSig_DSM_bRailMeUn2Blk  Interpolate=off  OutputAfterFinalValue=Holding final value
  spec_DSM_bRailMeUn2Rls : FromWorkspace  VariableName=testSig_DSM_bRailMeUn2Rls  Interpolate=off  OutputAfterFinalValue=Holding final value
  spec_DSM_bRailMeUn3Blk : FromWorkspace  VariableName=testSig_DSM_bRailMeUn3Blk  Interpolate=off  OutputAfterFinalValue=Holding final value
  spec_DSM_bRailMeUn3Rls : FromWorkspace  VariableName=testSig_DSM_bRailMeUn3Rls  Interpolate=off  OutputAfterFinalValue=Holding final value
  spec_DSM_bRailMeUn42Blk : FromWorkspace  VariableName=testSig_DSM_bRailMeUn42Blk  Interpolate=off  OutputAfterFinalValue=Holding final value
  spec_DSM_bRailMeUn42Rls : FromWorkspace  VariableName=testSig_DSM_bRailMeUn42Rls  Interpolate=off  OutputAfterFinalValue=Holding final value
  spec_DSM_bRailMeUn4Blk : FromWorkspace  VariableName=testSig_DSM_bRailMeUn4Blk  Interpolate=off  OutputAfterFinalValue=Holding final value
  spec_DSM_bRailMeUn4Rls : FromWorkspace  VariableName=testSig_DSM_bRailMeUn4Rls  Interpolate=off  OutputAfterFinalValue=Holding final value
  spec_DSM_bRailMeUn7Blk : FromWorkspace  VariableName=testSig_DSM_bRailMeUn7Blk  Interpolate=off  OutputAfterFinalValue=Holding final value
  spec_DSM_bRailMeUn7Rls : FromWorkspace  VariableName=testSig_DSM_bRailMeUn7Rls  Interpolate=off  OutputAfterFinalValue=Holding final value
  spec_DSM_bRailMeUn8Blk : FromWorkspace  VariableName=testSig_DSM_bRailMeUn8Blk  Interpolate=off  OutputAfterFinalValue=Holding final value
  spec_DSM_bRailMeUn8Rls : FromWorkspace  VariableName=testSig_DSM_bRailMeUn8Rls  Interpolate=off  OutputAfterFinalValue=Holding final value
  spec_Epm_nEng : FromWorkspace  VariableName=testSig_Epm_nEng  Interpolate=off  OutputAfterFinalValue=Holding final value
  spec_FuelT_tFlSys : FromWorkspace  VariableName=testSig_FuelT_tFlSys  Interpolate=off  OutputAfterFinalValue=Holding final value
  spec_InjCtl_qSetUnBal : FromWorkspace  VariableName=testSig_InjCtl_qSetUnBal  Interpolate=off  OutputAfterFinalValue=Holding final value
  spec_MeUn_dvolSet : FromWorkspace  VariableName=testSig_MeUn_dvolSet  Interpolate=off  OutputAfterFinalValue=Holding final value
  spec_MeUn_dvolSetAdapt : FromWorkspace  VariableName=testSig_MeUn_dvolSetAdapt  Interpolate=off  OutputAfterFinalValue=Holding final value
  spec_PthSet_stOvrRun : FromWorkspace  VariableName=testSig_PthSet_stOvrRun  Interpolate=off  OutputAfterFinalValue=Holding final value
  spec_RailP_pFlt : FromWorkspace  VariableName=testSig_RailP_pFlt  Interpolate=off  OutputAfterFinalValue=Holding final value
  spec_Rail_dvolDemSysMax : FromWorkspace  VariableName=testSig_Rail_dvolDemSysMax  Interpolate=off  OutputAfterFinalValue=Holding final value
  spec_Rail_dvolMeUnCtlUpLim : FromWorkspace  VariableName=testSig_Rail_dvolMeUnCtlUpLim  Interpolate=off  OutputAfterFinalValue=Holding final value
  spec_Rail_pDvt : FromWorkspace  VariableName=testSig_Rail_pDvt  Interpolate=off  OutputAfterFinalValue=Holding final value
  spec_Rail_pSetPoint : FromWorkspace  VariableName=testSig_Rail_pSetPoint  Interpolate=off  OutputAfterFinalValue=Holding final value
  spec_Rail_stCtlLoop : FromWorkspace  VariableName=testSig_Rail_stCtlLoop  Interpolate=off  OutputAfterFinalValue=Holding final value
  testSignals : Outport
  wires:
  BC/1 -> testSignals/1
  spec_Rail_pDvt/1 -> BC/1  "testSig_Rail_pDvt"
  spec_Epm_nEng/1 -> BC/2  "testSig_Epm_nEng"
  spec_MeUn_dvolSet/1 -> BC/3  "testSig_MeUn_dvolSet"
  spec_Rail_dvolMeUnCtlUpLim/1 -> BC/4  "testSig_Rail_dvolMeUnCtlUpLim"
  spec_Rail_stCtlLoop/1 -> BC/5  "testSig_Rail_stCtlLoop"
  spec_InjCtl_qSetUnBal/1 -> BC/6  "testSig_InjCtl_qSetUnBal"
  spec_FuelT_tFlSys/1 -> BC/7  "testSig_FuelT_tFlSys"
  spec_Rail_pSetPoint/1 -> BC/8  "testSig_Rail_pSetPoint"
  spec_Rail_dvolDemSysMax/1 -> BC/9  "testSig_Rail_dvolDemSysMax"
  spec_RailP_pFlt/1 -> BC/10  "testSig_RailP_pFlt"
  spec_MeUn_dvolSetAdapt/1 -> BC/11  "testSig_MeUn_dvolSetAdapt"
  spec_PthSet_stOvrRun/1 -> BC/12  "testSig_PthSet_stOvrRun"
  spec_APP_r/1 -> BC/13  "testSig_APP_r"
  spec_DSM_bRailMeUn0Rls/1 -> BC/14  "testSig_DSM_bRailMeUn0Rls"
  spec_DSM_bRailMeUn0Blk/1 -> BC/15  "testSig_DSM_bRailMeUn0Blk"
  spec_DSM_bRailMeUn2Rls/1 -> BC/16  "testSig_DSM_bRailMeUn2Rls"
  spec_DSM_bRailMeUn2Blk/1 -> BC/17  "testSig_DSM_bRailMeUn2Blk"
  spec_DSM_bRailMeUn22Rls/1 -> BC/18  "testSig_DSM_bRailMeUn22Rls"
  spec_DSM_bRailMeUn22Blk/1 -> BC/19  "testSig_DSM_bRailMeUn22Blk"
  spec_DSM_bRailMeUn3Rls/1 -> BC/20  "testSig_DSM_bRailMeUn3Rls"
  spec_DSM_bRailMeUn3Blk/1 -> BC/21  "testSig_DSM_bRailMeUn3Blk"
  spec_DSM_bRailMeUn4Rls/1 -> BC/22  "testSig_DSM_bRailMeUn4Rls"
  spec_DSM_bRailMeUn4Blk/1 -> BC/23  "testSig_DSM_bRailMeUn4Blk"
  spec_DSM_bRailMeUn42Rls/1 -> BC/24  "testSig_DSM_bRailMeUn42Rls"
  spec_DSM_bRailMeUn42Blk/1 -> BC/25  "testSig_DSM_bRailMeUn42Blk"
  spec_DSM_bRailMeUn7Rls/1 -> BC/26  "testSig_DSM_bRailMeUn7Rls"
  spec_DSM_bRailMeUn7Blk/1 -> BC/27  "testSig_DSM_bRailMeUn7Blk"
  spec_DSM_bRailMeUn8Rls/1 -> BC/28  "testSig_DSM_bRailMeUn8Rls"
  spec_DSM_bRailMeUn8Blk/1 -> BC/29  "testSig_DSM_bRailMeUn8Blk"
  spec_DSM_bRailMeUn10Rls/1 -> BC/30  "testSig_DSM_bRailMeUn10Rls"
  spec_DSM_bRailMeUn10Blk/1 -> BC/31  "testSig_DSM_bRailMeUn10Blk"
  spec_DFC_RailMeUn0_DSM/1 -> BC/32  "testSig_DFC_RailMeUn0_DSM"
  spec_DFC_RailMeUn2_DSM/1 -> BC/33  "testSig_DFC_RailMeUn2_DSM"
  spec_DFC_RailMeUn22_DSM/1 -> BC/34  "testSig_DFC_RailMeUn22_DSM"
  spec_DFC_RailMeUn3_DSM/1 -> BC/35  "testSig_DFC_RailMeUn3_DSM"
  spec_DFC_RailMeUn4_DSM/1 -> BC/36  "testSig_DFC_RailMeUn4_DSM"
  spec_DFC_RailMeUn42_DSM/1 -> BC/37  "testSig_DFC_RailMeUn42_DSM"
  spec_DFC_RailMeUn7_DSM/1 -> BC/38  "testSig_DFC_RailMeUn7_DSM"
  spec_DFC_RailMeUn8_DSM/1 -> BC/39  "testSig_DFC_RailMeUn8_DSM"
  spec_DFC_RailMeUn10_DSM/1 -> BC/40  "testSig_DFC_RailMeUn10_DSM"

== system TST_Rail_MonMeUn/compareSignals/Requirement_001/specifyOutputs ==
  sig_Req_Bus : Inport
  sig_Result_Bus : Inport  Port=2
  AndN : Logic  Inputs=9
  BS_Req : BusSelector  OutputSignals=testSig_DFC_RailMeUn0_DSM,testSig_DFC_RailMeUn2_DSM,testSig_DFC_RailMeUn22_DSM,testSig_DFC_RailMeUn3_DSM,testSig_DFC_RailMeUn4_DSM,testSig_DFC_RailMeUn42_DSM,testSig_DFC_RailMeUn7_DSM,testSig_DFC_RailMeUn8_DSM,testSig_DFC_RailMeUn10_DSM
  BS_Result : BusSelector  OutputSignals=DFC_RailMeUn0_DSM,DFC_RailMeUn2_DSM,DFC_RailMeUn22_DSM,DFC_RailMeUn3_DSM,DFC_RailMeUn4_DSM,DFC_RailMeUn42_DSM,DFC_RailMeUn7_DSM,DFC_RailMeUn8_DSM,DFC_RailMeUn10_DSM
  Bitwise_And{1..9} (9 alike) : simulink/Logic and Bit Operations/Bitwise Operator  logicop=AND  UseBitMask=off  BitMask=bin2dec('11011001')  BitMaskRealWorld=Stored Integer
  Scope : Scope  NumInputPorts=9
  Scope{1..9} (9 alike) : Scope  NumInputPorts=2
  cmp_{1..9} (9 alike) : UnitTest_Lib/RoughlyEqual  slope=0.1
  result_tws : ToWorkspace  VariableName=spec_result_001
  tws_1 : ToWorkspace  VariableName=spec_req_001_001
  tws_2 : ToWorkspace  VariableName=spec_req_001_002
  tws_3 : ToWorkspace  VariableName=spec_req_001_003
  tws_4 : ToWorkspace  VariableName=spec_req_001_004
  tws_5 : ToWorkspace  VariableName=spec_req_001_005
  tws_6 : ToWorkspace  VariableName=spec_req_001_006
  tws_7 : ToWorkspace  VariableName=spec_req_001_007
  tws_8 : ToWorkspace  VariableName=spec_req_001_008
  tws_9 : ToWorkspace  VariableName=spec_req_001_009
  result : Outport
  wires:
  sig_Req_Bus/1 -> BS_Req/1
  sig_Result_Bus/1 -> BS_Result/1
  AndN/1 -> result/1, result_tws/1
  BS_Req/1 -> cmp_1/1, Scope1/1  "<testSig_DFC_RailMeUn0_DSM>"
  BS_Result/1 -> cmp_1/2, Scope1/2  "<DFC_RailMeUn0_DSM>"
  cmp_1/1 -> Bitwise_And1/1
  Bitwise_And1/1 -> tws_1/1, AndN/1, Scope/1
  BS_Req/2 -> cmp_2/1, Scope2/1  "<testSig_DFC_RailMeUn2_DSM>"
  BS_Result/2 -> cmp_2/2, Scope2/2  "<DFC_RailMeUn2_DSM>"
  cmp_2/1 -> Bitwise_And2/1
  Bitwise_And2/1 -> tws_2/1, AndN/2, Scope/2
  BS_Req/3 -> cmp_3/1, Scope3/1  "<testSig_DFC_RailMeUn22_DSM>"
  BS_Result/3 -> cmp_3/2, Scope3/2  "<DFC_RailMeUn22_DSM>"
  cmp_3/1 -> Bitwise_And3/1
  Bitwise_And3/1 -> tws_3/1, AndN/3, Scope/3
  BS_Req/4 -> cmp_4/1, Scope4/1  "<testSig_DFC_RailMeUn3_DSM>"
  BS_Result/4 -> cmp_4/2, Scope4/2  "<DFC_RailMeUn3_DSM>"
  cmp_4/1 -> Bitwise_And4/1
  Bitwise_And4/1 -> tws_4/1, AndN/4, Scope/4
  BS_Req/5 -> cmp_5/1, Scope5/1  "<testSig_DFC_RailMeUn4_DSM>"
  BS_Result/5 -> cmp_5/2, Scope5/2  "<DFC_RailMeUn4_DSM>"
  cmp_5/1 -> Bitwise_And5/1
  Bitwise_And5/1 -> tws_5/1, AndN/5, Scope/5
  BS_Req/6 -> cmp_6/1, Scope6/1  "<testSig_DFC_RailMeUn42_DSM>"
  BS_Result/6 -> cmp_6/2, Scope6/2  "<DFC_RailMeUn42_DSM>"
  cmp_6/1 -> Bitwise_And6/1
  Bitwise_And6/1 -> tws_6/1, AndN/6, Scope/6
  BS_Req/7 -> cmp_7/1, Scope7/1  "<testSig_DFC_RailMeUn7_DSM>"
  BS_Result/7 -> cmp_7/2, Scope7/2  "<DFC_RailMeUn7_DSM>"
  cmp_7/1 -> Bitwise_And7/1
  Bitwise_And7/1 -> tws_7/1, AndN/7, Scope/7
  BS_Req/8 -> cmp_8/1, Scope8/1  "<testSig_DFC_RailMeUn8_DSM>"
  BS_Result/8 -> cmp_8/2, Scope8/2  "<DFC_RailMeUn8_DSM>"
  cmp_8/1 -> Bitwise_And8/1
  Bitwise_And8/1 -> tws_8/1, AndN/8, Scope/8
  BS_Req/9 -> cmp_9/1, Scope9/1  "<testSig_DFC_RailMeUn10_DSM>"
  BS_Result/9 -> cmp_9/2, Scope9/2  "<DFC_RailMeUn10_DSM>"
  cmp_9/1 -> Bitwise_And9/1
  Bitwise_And9/1 -> tws_9/1, AndN/9, Scope/9

== system TST_Rail_MonMeUn/compareSignals/Requirement_002/specifyOutputs ==
  sig_Req_Bus : Inport
  sig_Result_Bus : Inport  Port=2
  AndN : Logic  Inputs=9
  BS_Req : BusSelector  OutputSignals=testSig_DFC_RailMeUn0_DSM,testSig_DFC_RailMeUn2_DSM,testSig_DFC_RailMeUn22_DSM,testSig_DFC_RailMeUn3_DSM,testSig_DFC_RailMeUn4_DSM,testSig_DFC_RailMeUn42_DSM,testSig_DFC_RailMeUn7_DSM,testSig_DFC_RailMeUn8_DSM,testSig_DFC_RailMeUn10_DSM
  BS_Result : BusSelector  OutputSignals=DFC_RailMeUn0_DSM,DFC_RailMeUn2_DSM,DFC_RailMeUn22_DSM,DFC_RailMeUn3_DSM,DFC_RailMeUn4_DSM,DFC_RailMeUn42_DSM,DFC_RailMeUn7_DSM,DFC_RailMeUn8_DSM,DFC_RailMeUn10_DSM
  Bitwise_And{1..9} (9 alike) : simulink/Logic and Bit Operations/Bitwise Operator  logicop=AND  UseBitMask=off  BitMask=bin2dec('11011001')  BitMaskRealWorld=Stored Integer
  Scope : Scope  NumInputPorts=9
  Scope{1..9} (9 alike) : Scope  NumInputPorts=2
  cmp_{1..9} (9 alike) : UnitTest_Lib/RoughlyEqual  slope=0.1
  result_tws : ToWorkspace  VariableName=spec_result_002
  tws_1 : ToWorkspace  VariableName=spec_req_002_001
  tws_2 : ToWorkspace  VariableName=spec_req_002_002
  tws_3 : ToWorkspace  VariableName=spec_req_002_003
  tws_4 : ToWorkspace  VariableName=spec_req_002_004
  tws_5 : ToWorkspace  VariableName=spec_req_002_005
  tws_6 : ToWorkspace  VariableName=spec_req_002_006
  tws_7 : ToWorkspace  VariableName=spec_req_002_007
  tws_8 : ToWorkspace  VariableName=spec_req_002_008
  tws_9 : ToWorkspace  VariableName=spec_req_002_009
  result : Outport
  wires:
  sig_Req_Bus/1 -> BS_Req/1
  sig_Result_Bus/1 -> BS_Result/1
  AndN/1 -> result/1, result_tws/1
  BS_Req/1 -> cmp_1/1, Scope1/1  "<testSig_DFC_RailMeUn0_DSM>"
  BS_Result/1 -> cmp_1/2, Scope1/2  "<DFC_RailMeUn0_DSM>"
  cmp_1/1 -> Bitwise_And1/1
  Bitwise_And1/1 -> tws_1/1, AndN/1, Scope/1
  BS_Req/2 -> cmp_2/1, Scope2/1  "<testSig_DFC_RailMeUn2_DSM>"
  BS_Result/2 -> cmp_2/2, Scope2/2  "<DFC_RailMeUn2_DSM>"
  cmp_2/1 -> Bitwise_And2/1
  Bitwise_And2/1 -> tws_2/1, AndN/2, Scope/2
  BS_Req/3 -> cmp_3/1, Scope3/1  "<testSig_DFC_RailMeUn22_DSM>"
  BS_Result/3 -> cmp_3/2, Scope3/2  "<DFC_RailMeUn22_DSM>"
  cmp_3/1 -> Bitwise_And3/1
  Bitwise_And3/1 -> tws_3/1, AndN/3, Scope/3
  BS_Req/4 -> cmp_4/1, Scope4/1  "<testSig_DFC_RailMeUn3_DSM>"
  BS_Result/4 -> cmp_4/2, Scope4/2  "<DFC_RailMeUn3_DSM>"
  cmp_4/1 -> Bitwise_And4/1
  Bitwise_And4/1 -> tws_4/1, AndN/4, Scope/4
  BS_Req/5 -> cmp_5/1, Scope5/1  "<testSig_DFC_RailMeUn4_DSM>"
  BS_Result/5 -> cmp_5/2, Scope5/2  "<DFC_RailMeUn4_DSM>"
  cmp_5/1 -> Bitwise_And5/1
  Bitwise_And5/1 -> tws_5/1, AndN/5, Scope/5
  BS_Req/6 -> cmp_6/1, Scope6/1  "<testSig_DFC_RailMeUn42_DSM>"
  BS_Result/6 -> cmp_6/2, Scope6/2  "<DFC_RailMeUn42_DSM>"
  cmp_6/1 -> Bitwise_And6/1
  Bitwise_And6/1 -> tws_6/1, AndN/6, Scope/6
  BS_Req/7 -> cmp_7/1, Scope7/1  "<testSig_DFC_RailMeUn7_DSM>"
  BS_Result/7 -> cmp_7/2, Scope7/2  "<DFC_RailMeUn7_DSM>"
  cmp_7/1 -> Bitwise_And7/1
  Bitwise_And7/1 -> tws_7/1, AndN/7, Scope/7
  BS_Req/8 -> cmp_8/1, Scope8/1  "<testSig_DFC_RailMeUn8_DSM>"
  BS_Result/8 -> cmp_8/2, Scope8/2  "<DFC_RailMeUn8_DSM>"
  cmp_8/1 -> Bitwise_And8/1
  Bitwise_And8/1 -> tws_8/1, AndN/8, Scope/8
  BS_Req/9 -> cmp_9/1, Scope9/1  "<testSig_DFC_RailMeUn10_DSM>"
  BS_Result/9 -> cmp_9/2, Scope9/2  "<DFC_RailMeUn10_DSM>"
  cmp_9/1 -> Bitwise_And9/1
  Bitwise_And9/1 -> tws_9/1, AndN/9, Scope/9
